simulink model "rassim"  (R2020b)
settings: Solver=VariableStepAuto  StartTime=0.0  StopTime=5  RelTol=1e-3
values from neighbouring files (symbols this model uses):
  d2x = sym('d2x', 'real')    [AL.m]    (also in FL.m; main.m = 0)
  d2z = sym('d2z', 'real')    [AL.m]    (also in FL.m; main.m = 0.0979)
  dgx = sym('dgx', 'real')    [AL.m]    (also in FL.m; main.m = 0)
  gravity = sym('gravity','real')    [AL.m]    (also in FL.m; main.m = 9.81)
  J1 = sym('J1', 'real')    [AL.m]    (also in FL.m; main.m = 0.0154)
  J2 = sym('J2', 'real')    [AL.m]    (also in FL.m; main.m = 0.0011)
  Jm = sym('Jm', 'real')    [AL.m]    (also in FL.m; main.m = 0.4101)
  m1 = sym('m1','real')    [AL.m]    (also in FL.m; main.m = 1.309)
  m2 = sym('m2','real')    [AL.m]    (also in FL.m; main.m = 0.098)
  mM = sym('mM','real')    [AL.m]    (also in FL.m = sym('m','real'); main.m = 0.06)
settings Model: Creator=Tommaso  LastModifiedBy=Tommaso
settings DataIOCC: ReturnWorkspaceOutputs=off

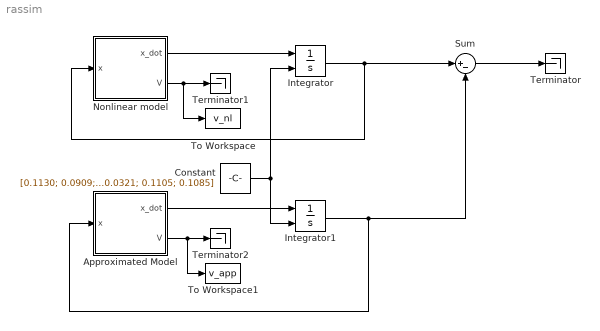
== system rassim ==
  Approximated Model : MATLAB Function  TreatAsAtomicUnit=on
  Constant : Constant  Value=|
      | [0.1130;
      | 0.0909;
      | -0.1556;
      | 0.2625;
      | -0.1362;
      | 0.0321;
      | 0.1105;
      | 0.1085]
  Integrator : Integrator  InitialConditionSource=external  InitialCondition=[0; 0; 0; 0; 0; 0; 0; 0]
  Integrator1 : Integrator  InitialConditionSource=external  InitialCondition=[0; 0; 0; 0; 0; 0; 0; 0]
  Nonlinear model : MATLAB Function  TreatAsAtomicUnit=on
  Sum : Sum  Inputs=|+-
  Terminator : Terminator
  Terminator1 : Terminator
  Terminator2 : Terminator
  To Workspace : ToWorkspace  VariableName=v_nl  SaveFormat=Timeseries  SampleTime=-1
  To Workspace1 : ToWorkspace  VariableName=v_app  SaveFormat=Timeseries  SampleTime=-1
  wires:
  Nonlinear model/1(x_dot) -> Integrator/1
  Approximated Model/1(x_dot) -> Integrator1/1
  Sum/1 -> Terminator/1
  Integrator/1 -> Nonlinear model/1(x), Sum/1
  Integrator1/1 -> Approximated Model/1(x), Sum/2
  Constant/1 -> Integrator1/2, Integrator/2
  Nonlinear model/2(V) -> To Workspace/1, Terminator1/1
  Approximated Model/2(V) -> To Workspace1/1, Terminator2/1

== matlab function rassim/Nonlinear model ==
  data: x input; x_dot output; m1 parameter; m2 parameter; mM parameter; J1 parameter; J2 parameter; Jm parameter; d2x parameter; d2z parameter; dgx parameter; gravity parameter; V output
function [x_dot, V] = model(x, m1, m2, mM, J1, J2, Jm, d2x, d2z, dgx, gravity)

% State variables
pc1x = x(1);
pc1z = x(2);
pc1x_dot = x(3);
pc1z_dot = x(4);
theta1 = x(5);
theta1_dot = x(6);
theta12 = x(7);
theta12_dot = x(8);

% Parameters
d2 = [d2x; d2z];
beta1 = -m2*(d2x*cos(theta12) + d2z*sin(theta12));
beta2 = -m2*(d2z*cos(theta12) - d2x*sin(theta12));
g4 = m2*gravity*(d2x*cos(theta12) + d2z*sin(theta12));
mb = J2 + Jm + m2*norm(d2)^2;
ms = m1 + m2 + mM;

% Dynamic matrices
g = [0; -ms*gravity; 0; g4];
C = [beta1*theta12_dot^2; beta2*theta12_dot^2; 0; 0];
M = [ms 0 0 beta1; 0 ms 0 beta2; 0 0 J1 0; beta1 beta2 0 mb];
G = [-sin(theta1) 0 0; -cos(theta1) 0 0; dgx 1 -1; 0 0 1];

x = [pc1x, pc1z, pc1x_dot, pc1z_dot, theta1, theta1_dot, theta12, theta12_dot]';

% State space representation
x1_dot = x(3);
x2_dot = x(4);
x5_dot = x(6);
x7_dot = x(8);

q_ddot = (inv(M))*(-C - g);
x3_dot = q_ddot(1);
x4_dot = q_ddot(2);
x6_dot = q_ddot(3);
x8_dot = q_ddot(4);

% Drift field (8x1)
f_x = [x1_dot; x2_dot; x3_dot; x4_dot; x5_dot; x6_dot; x7_dot; x8_dot];

% Control field (8x3)
invMG = (inv(M))*G;
g_x = [0 0 0; 0 0 0; invMG(1,:); invMG(2,:); 0 0 0; invMG(3,:); 0 0 0; invMG(4,:)];

u_eq = [                     gravity*(m1 + m2 + mM)
        d2x*gravity*m2 - dgx*gravity*(m1 + m2 + mM)
                                    d2x*gravity*m2];

% Affine-form system
% K = [   11.8868  -34.1978   13.9820  -14.7309  -40.2201   -3.3316   -9.0103   -1.8396
%          2.3946    2.9691    2.8254    0.5751   -8.2740   -0.5848    7.3219    3.7592
%          2.5781    2.9524    3.1255    0.5720   -9.6981   -0.8432    7.3350    3.7601];
K = [    
   -0.0317   -8.8016   -0.0244   -7.6099    0.0806    0.0134   -3.5832   -1.4245
   -0.0270    1.0114   -0.0707    0.4091    0.4460    0.1586    1.9661    1.9835
    0.0107    1.0114    0.0078    0.4091   -0.0930    0.0046    1.9659    1.9830];

u = -K*x + u_eq;

x_dot = f_x + g_x*u;

P = [1.7500         0    0.9700         0   -2.4100   -0.2000         0   -0.0100
         0    1.1400         0    0.1000         0         0   -0.0200   -0.0500
    0.9700         0    1.2900         0   -3.4400   -0.2900   -0.0100   -0.0100
         0    0.1000         0    0.1200         0         0   -0.0500   -0.0400
   -2.4100         0   -3.4400         0   12.1200    0.9800    0.0100    0.0200
   -0.2000         0   -0.2900         0    0.9800    0.1500         0         0
         0   -0.0200   -0.0100   -0.0500    0.0100         0    1.1500    0.1300
   -0.0100   -0.0500   -0.0100   -0.0400    0.0200         0    0.1300    0.1400];

V = x'*P*x;

== matlab function rassim/Approximated Model ==
  data: x input; x_dot output; m1 parameter; m2 parameter; mM parameter; J1 parameter; J2 parameter; Jm parameter; d2x parameter; d2z parameter; dgx parameter; gravity parameter; V output
function [x_dot, V] = model(x, m1, m2, mM, J1, J2, Jm, d2x, d2z, dgx, gravity)

% State variables
pc1x = x(1);
pc1z = x(2);
pc1x_dot = x(3);
pc1z_dot = x(4);
theta1 = x(5);
theta1_dot = x(6);
theta12 = x(7);
theta12_dot = x(8);

% Parameters

x = [pc1x, pc1z, pc1x_dot, pc1z_dot, theta1, theta1_dot, theta12, theta12_dot]';

u_eq = [                     gravity*(m1 + m2 + mM)
        d2x*gravity*m2 - dgx*gravity*(m1 + m2 + mM)
                                    d2x*gravity*m2];

A = [0, 0, 1, 0,                                                                                                                                                                                                                                       0, 0,                                                                                                                                                                                                                                                                                                                                                                                                                                                                                0, 0
     0, 0, 0, 1,                                                                                                                                                                                                                                       0, 0,                                                                                                                                                                                                                                                                                                                                                                                                                                                                                0, 0
     0, 0, 0, 0, -(gravity*(J2*m1 + J2*m2 + J2*mM + Jm*m1 + Jm*m2 + Jm*mM + d2z^2*m2^2 + d2x^2*m1*m2 + d2z^2*m1*m2 + d2x^2*m2*mM + d2z^2*m2*mM))/(J2*m1 + J2*m2 + J2*mM + Jm*m1 + Jm*m2 + Jm*mM + d2x^2*m1*m2 + d2z^2*m1*m2 + d2x^2*m2*mM + d2z^2*m2*mM), 0, (gravity*(d2x^2*m2^2 - d2z^2*m2^2))/(J2*m1 + J2*m2 + J2*mM + Jm*m1 + Jm*m2 + Jm*mM + d2x^2*m1*m2 + d2z^2*m1*m2 + d2x^2*m2*mM + d2z^2*m2*mM) - (2*d2x^2*gravity*m2^3 + 2*d2x^2*gravity*m1*m2^2 + 2*d2x^2*gravity*m2^2*mM)/((m1 + m2 + mM)*(J2*m1 + J2*m2 + J2*mM + Jm*m1 + Jm*m2 + Jm*mM + d2x^2*m1*m2 + d2z^2*m1*m2 + d2x^2*m2*mM + d2z^2*m2*mM)) + (d2x^2*gravity*m2^2)/(J2*m1 + J2*m2 + J2*mM + Jm*m1 + Jm*m2 + Jm*mM + d2x^2*m1*m2 + d2z^2*m1*m2 + d2x^2*m2*mM + d2z^2*m2*mM), 0
     0, 0, 0, 0,                                                                                                          (d2x*d2z*gravity*m2^2)/(J2*m1 + J2*m2 + J2*mM + Jm*m1 + Jm*m2 + Jm*mM + d2x^2*m1*m2 + d2z^2*m1*m2 + d2x^2*m2*mM + d2z^2*m2*mM), 0,                                                                                                                                     (3*d2x*d2z*gravity*m2^2)/(J2*m1 + J2*m2 + J2*mM + Jm*m1 + Jm*m2 + Jm*mM + d2x^2*m1*m2 + d2z^2*m1*m2 + d2x^2*m2*mM + d2z^2*m2*mM) - (2*d2x*d2z*gravity*m2^3 + 2*d2x*d2z*gravity*m1*m2^2 + 2*d2x*d2z*gravity*m2^2*mM)/((m1 + m2 + mM)*(J2*m1 + J2*m2 + J2*mM + Jm*m1 + Jm*m2 + Jm*mM + d2x^2*m1*m2 + d2z^2*m1*m2 + d2x^2*m2*mM + d2z^2*m2*mM)), 0
     0, 0, 0, 0,                                                                                                                                                                                                                                       0, 1,                                                                                                                                                                                                                                                                                                                                                                                                                                                                                0, 0
     0, 0, 0, 0,                                                                                                                                                                                                                                       0, 0,                                                                                                                                                                                                                                                                                                                                                                                                                                                                                0, 0
     0, 0, 0, 0,                                                                                                                                                                                                                                       0, 0,                                                                                                                                                                                                                                                                                                                                                                                                                                                                                0, 1
     0, 0, 0, 0,                                                                                                -(d2z*gravity*m2*(m1 + m2 + mM))/(J2*m1 + J2*m2 + J2*mM + Jm*m1 + Jm*m2 + Jm*mM + d2x^2*m1*m2 + d2z^2*m1*m2 + d2x^2*m2*mM + d2z^2*m2*mM), 0,                                                                                                                                                                                                                                                                                                                                         -(d2z*gravity*m2*(m1 + m2 + mM))/(J2*m1 + J2*m2 + J2*mM + Jm*m1 + Jm*m2 + Jm*mM + d2x^2*m1*m2 + d2z^2*m1*m2 + d2x^2*m2*mM + d2z^2*m2*mM), 0];


 
B = [                                                                                                                                                                                                                                             0,    0,                                                                                                                     0
                                                                                                                                                                                                                                                 0,    0,                                                                                                                      0
                                                                                                           (d2x*d2z*m2^2)/((m1 + m2 + mM)*(J2*m1 + J2*m2 + J2*mM + Jm*m1 + Jm*m2 + Jm*mM + d2x^2*m1*m2 + d2z^2*m1*m2 + d2x^2*m2*mM + d2z^2*m2*mM)),    0,       (d2z*m2)/(J2*m1 + J2*m2 + J2*mM + Jm*m1 + Jm*m2 + Jm*mM + d2x^2*m1*m2 + d2z^2*m1*m2 + d2x^2*m2*mM + d2z^2*m2*mM)
    -(J2*m1 + J2*m2 + J2*mM + Jm*m1 + Jm*m2 + Jm*mM + d2x^2*m2^2 + d2x^2*m1*m2 + d2z^2*m1*m2 + d2x^2*m2*mM + d2z^2*m2*mM)/((m1 + m2 + mM)*(J2*m1 + J2*m2 + J2*mM + Jm*m1 + Jm*m2 + Jm*mM + d2x^2*m1*m2 + d2z^2*m1*m2 + d2x^2*m2*mM + d2z^2*m2*mM)),    0,      -(d2x*m2)/(J2*m1 + J2*m2 + J2*mM + Jm*m1 + Jm*m2 + Jm*mM + d2x^2*m1*m2 + d2z^2*m1*m2 + d2x^2*m2*mM + d2z^2*m2*mM)
                                                                                                                                                                                                                                                 0,    0,                                                                                                                      0
                                                                                                                                                                                                                                            dgx/J1, 1/J1,                                                                                                                  -1/J1
                                                                                                                                                                                                                                                 0,    0,                                                                                                                      0
                                                                                                                                  (d2x*m2)/(J2*m1 + J2*m2 + J2*mM + Jm*m1 + Jm*m2 + Jm*mM + d2x^2*m1*m2 + d2z^2*m1*m2 + d2x^2*m2*mM + d2z^2*m2*mM),    0, (m1 + m2 + mM)/(J2*m1 + J2*m2 + J2*mM + Jm*m1 + Jm*m2 + Jm*mM + d2x^2*m1*m2 + d2z^2*m1*m2 + d2x^2*m2*mM + d2z^2*m2*mM)];
                                                                                                                              
% K = [   11.8868  -34.1978   13.9820  -14.7309  -40.2201   -3.3316   -9.0103   -1.8396
%          2.3946    2.9691    2.8254    0.5751   -8.2740   -0.5848    7.3219    3.7592
%          2.5781    2.9524    3.1255    0.5720   -9.6981   -0.8432    7.3350    3.7601];
K = [
   -0.0317   -8.8016   -0.0244   -7.6099    0.0806    0.0134   -3.5832   -1.4245
   -0.0270    1.0114   -0.0707    0.4091    0.4460    0.1586    1.9661    1.9835
    0.0107    1.0114    0.0078    0.4091   -0.0930    0.0046    1.9659    1.9830];


u = -K*x + u_eq;
x_dot = A*x + B*(u - u_eq); 

P = [1.7500         0    0.9700         0   -2.4100   -0.2000         0   -0.0100
         0    1.1400         0    0.1000         0         0   -0.0200   -0.0500
    0.9700         0    1.2900         0   -3.4400   -0.2900   -0.0100   -0.0100
         0    0.1000         0    0.1200         0         0   -0.0500   -0.0400
   -2.4100         0   -3.4400         0   12.1200    0.9800    0.0100    0.0200
   -0.2000         0   -0.2900         0    0.9800    0.1500         0         0
         0   -0.0200   -0.0100   -0.0500    0.0100         0    1.1500    0.1300
   -0.0100   -0.0500   -0.0100   -0.0400    0.0200         0    0.1300    0.1400];

V = x'*P*x;
